simulink model "joystickdemo"  (R2025a)
settings: Solver=VariableStepAuto  StartTime=0.0  StopTime=t_final  RelTol=1e-3
values from neighbouring files (symbols this model uses):
  dt = 1/50    (= 0.02)    [InitializeConstants.m]    (also in joystickdemo.m)
libraries: aerolibanimutils x2
settings Model: PauseTimes=t_final  Creator=pjpra  LastModifiedBy=pjpra

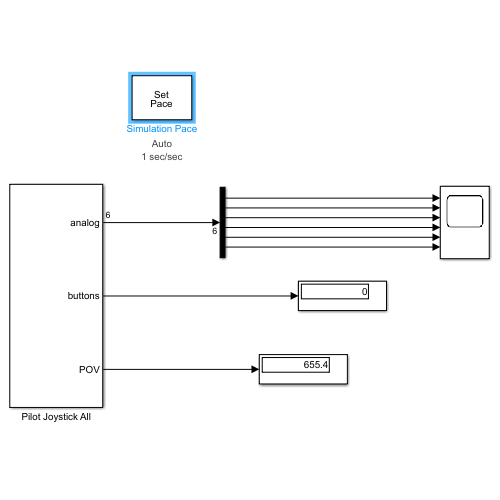
[thumbnail: Simulink's stored preview of the top-level diagram]
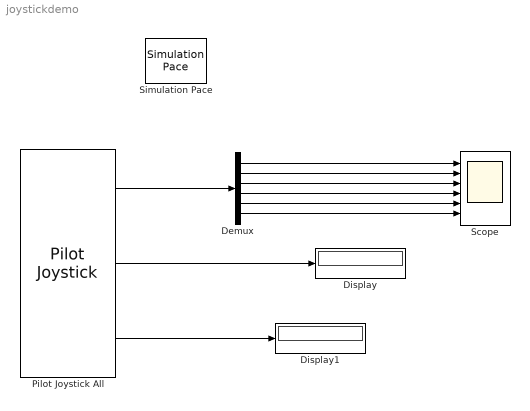
== system joystickdemo ==
  Demux : Demux  Outputs=6
  Display : Display
  Display1 : Display
  Pilot Joystick All : aerolibanimutils/Pilot Joystick  JoystickID=Joystick1  OutputConfiguration=AllOutputs  SampleTime=dt
      settings: LibrarySourceBlock=aerolibanimutils/Pilot Joystick All
  Scope : Scope  NumInputPorts=6
  Simulation Pace : aerolibanimutils/Simulation Pace  SimulationPace=1  SleepMode=Auto  OutputPaceError=off  SampleTime=dt
  wires:
  Pilot Joystick All/1 -> Demux/1
  Pilot Joystick All/2 -> Display/1
  Pilot Joystick All/3 -> Display1/1
  Demux/3 -> Scope/3
  Demux/2 -> Scope/2
  Demux/1 -> Scope/1
  Demux/4 -> Scope/4
  Demux/5 -> Scope/5
  Demux/6 -> Scope/6
